simulink model "simu_25a"  (R2025a)
settings: Solver=VariableStepAuto  StartTime=0.0  StopTime=0.5  RelTol=1e-3
settings Model: Creator=psp_dada  LastModifiedBy=psp_dada

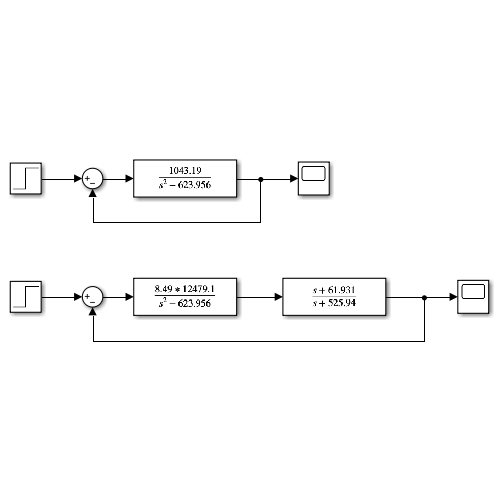
[thumbnail: Simulink's stored preview of the top-level diagram]
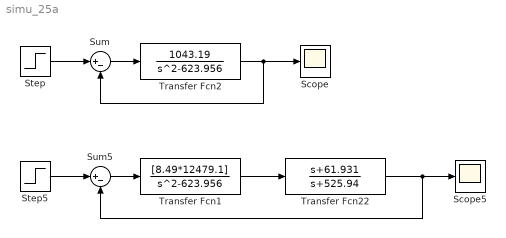
== system simu_25a ==
  Scope : Scope
      settings: ActiveDisplayYMinimum=-1  ActiveDisplayYMaximum=1
  Scope5 : Scope
      settings: ActiveDisplayYMinimum=-0.1599  ActiveDisplayYMaximum=1.43906
  Step : Step  SampleTime=0
  Step5 : Step  Time=0.1  SampleTime=0
  Sum : Sum  Inputs=|+-
  Sum5 : Sum  Inputs=|+-
  Transfer Fcn1 : TransferFcn  Numerator=[8.49*12479.1]  Denominator=[1 0 -623.956]
  Transfer Fcn2 : TransferFcn  Numerator=[1043.19]  Denominator=[1 0 -623.956]
  Transfer Fcn22 : TransferFcn  Numerator=[1 61.931]  Denominator=[1 525.94]
  wires:
  Step/1 -> Sum/1
  Sum/1 -> Transfer Fcn2/1
  Transfer Fcn2/1 -> Scope/1, Sum/2
  Sum5/1 -> Transfer Fcn1/1
  Step5/1 -> Sum5/1
  Transfer Fcn1/1 -> Transfer Fcn22/1
  Transfer Fcn22/1 -> Scope5/1, Sum5/2
